simulink model "Simplified_TriPed"  (R2020a)
settings: Solver=VariableStepAuto  StartTime=0.0  StopTime=inf  RelTol=1e-3  EnableMultiTasking=on
values from neighbouring files (symbols this model uses):
  s = 1/(2*r)    [Weg0.m]
undefined symbols (not defined in the file or in its folder): sigbuilder_block, X, Y, Z
libraries: sm_lib x13, nesl_utility x4, ros2lib x3, powerlib_meascontrol x3, simulink x2, vrlib x1
(part 1 of 2)
settings Model: PacingRate=0.100000  OrderedModelArguments=off  Creator=maxde  LastModifiedBy=jan-b
settings DataIOCC: LimitDataPoints=on  MaxDataPoints=10000
settings OptimizationCC: LifeSpan=inf
settings DebuggingCC: AllowSymbolicDim=off  SFUnexpectedBacktrackingDiag=warning  SFNoUnconditionalDefaultTransitionDiag=warning  SFExecutionAtInitializationDiag=none  ArithmeticOperatorsInVariantConditions=warning
settings SFSimCC: SimUseLocalCustomCode=off  CustomCodeUndefinedFunction=UseInterfaceOnly
settings RTWCC: RTWUseLocalCustomCode=off
settings CodeAppCC: StateflowObjectComments=on
settings GRTTargetCC: TargetLangStandard=C89/C90 (ANSI)
settings ConfigComp: CovMetricSettings=dw  CovHtmlReporting=on  CovSaveCumulativeToWorkspaceVar=on  CovSaveSingleToWorkspaceVar=on  CovExternalEMLEnable=off  CovSFcnEnable=off
settings SimscapeCC: SimscapeLogType=all  SimscapeLogSimulationStatistics=on  SimscapeLogDataHistory=10000

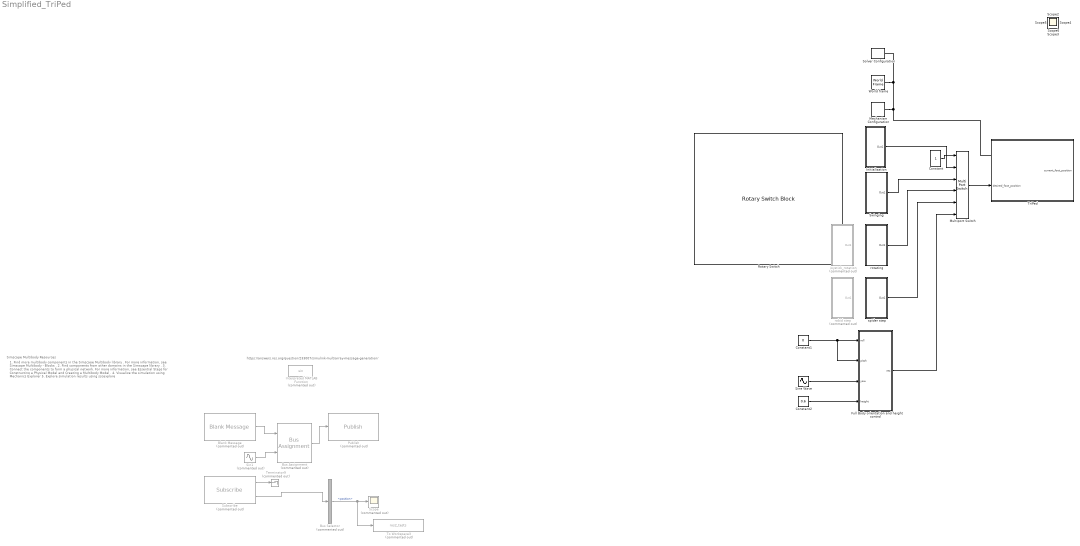
== system Simplified_TriPed ==
  note: https://answers.ros.org/question/233007/simulink-multiarray-message-generation/
  note: 1. Find more multibody components in the Simscape Multibody library .
      | For more information, see Simscape Multibody - Blocks .
      | 2. Find components from other domains in the Simscape library .
      | 3. Connect the components to form a physical network.
      | For more information, see Essential Steps for Constructing a Physical Model and Creating a Multibody Model .
      | 4. Visualize the simulation using Mechanics Explorer
      | 5. Explore simulation results using sscexplore
  note: Simscape Multibody Resources
  Blank Message : ros2lib/Blank Message  Commented=on  messageType=pendulum_msgs/JointState  SampleTime=inf
      settings: SourceProductBaseCode=RR
  Bus Assignment : BusAssignment  Commented=on  AssignedSignals=position
  Bus Selector : BusSelector  Commented=on  OutputSignals=position
  Constant : Constant
  Constant1 : Constant  Value=0
  Constant2 : Constant  Value=0.6
  Full Body orientation and height control : Subsystem
  Initialisation : Subsystem
  Interpreted MATLAB Function : MATLABFcn  Commented=on
  Mechanism Configuration : sm_lib/Utilities/Mechanism Configuration  UniformGravity=Constant  GravityVector=[0 0 -9.80665]  GravityUnits=m/s^2  LinearizationDelta=0.001
  Multiport Switch : MultiPortSwitch  Inputs=5
  Publish : ros2lib/Publish  Commented=on  topicSource=Specify your own  topic=/test_geometry  messageType=pendulum_msgs/JointState  QOSHistory=Keep last  QOSDepth=1  QOSReliability=Reliable  QOSDurability=Volatile
      settings: SourceProductBaseCode=RR
  Rotary Switch : RotarySwitchBlock
      settings: Values={{'Initialisation', 'Swinging', 'Rotating', 'Stepping', 'Full Body Kinematics'}, [1 2 3 4 5]}
  Scope : Scope  Commented=on
  Sin1 : Sin  Commented=on  Amplitude=pi/4  Frequency=2*pi/1  SampleTime=0.02
  Sine Wave : Sin  SampleTime=0
  Solver Configuration : nesl_utility/Solver Configuration  PhysicalDomain=network_engine_domain  SubClassName=solver  LeftPortType=input  RightPortType=generic  Tones=[]  Harmonics=[]  SimulateNoise=off  Profile=off  UseLocalSampling=off  EnableSwitchedLinearOptims=on  FrequencyDomain=off  UseCCode=off  RelTol=0.001  AbsTol=1e-06  MinStep=1e-09  ToWorkspace=off  RevertToSquareIcSolve=off  NumHomotopyIterations=100  PhasorMode=off  PhasorModeNumHarmonics=1  DoDC=off  ResidualTolerance=1e-09  UseLocalSolver=off  LocalSolverChoice=NE_BACKWARD_EULER_ADVANCER  LocalSolverSampleTime=0.001  DoFixedCost=off  MaxNonlinIter=3  MaxModeIter=2  LinearAlgebra=Sparse  EquationFormulation=NE_TIME_EF  DelaysMemoryBudget=1024  AutomaticFiltering=on  FilteringTimeConstant=0.001  PartitionStorageMethod=AS_NEEDED  PartitionMemoryBudget=1024  PartitionMethod=FAST
      settings: SourceProductBaseCode=MT,SS
  Subscribe : ros2lib/Subscribe  Commented=on  topicSource=Specify your own  topic=/test_geometry  messageType=pendulum_msgs/JointState  sampleTime=-1  QOSHistory=Keep last  QOSDepth=1  QOSReliability=Reliable  QOSDurability=Volatile
      settings: SourceProductBaseCode=RR
  Swinging : Subsystem
  Terminator9 : Terminator  Commented=on
  To Workspace3 : ToWorkspace  Commented=on  VariableName=ros2_tests  SaveFormat=Timeseries  SampleTime=-1
  TriPed : Subsystem
      settings: PortSchema="{\"entries\":[{\"content\":{\"sides\":[{\"content\":{\"connectorIds\":[\"LConn1\",\"In1\"]},\"type\":\"ConnectorPlacement.EquallySpacedRectSide\",\"uuid\":\"cf937cc4-9946-458f-a00c-c6b64d50e5dd\"},{\"content\":{\"connectorIds\":[\"Out1\"],\"side\":\"RIGHT\"},\"type\":\"ConnectorPlacement.EquallySpacedRectSide\",\"uuid\":\"24e17f8e-a145-44bf-b20e-4a80bbb5751f\"},{\"content\":{\"connectorIds\":[],\"side\":\"TOP\"},\"type\":\"ConnectorPlacement.EquallySpacedRectSide\",\"uuid\":\"6e43fe6c-017a-4e02-a518-41141b50f8f7\"}]},\"type\":\"ConnectorPlacement.EquallySpacedConnector\",\"uuid\":\"8dc904d1-a5ef-4597-b7a1-5eba3e01f89e\"}],\"packageUris\":[\"http://schema.mathworks.com/mf0/Connector/19700101\"],\"version\":\"1.0\"}"
      mask Display: image('./icons/triped_complete_view.png')
  World frame : sm_lib/Frames and Transforms/World Frame
  joystick_rotation : Subsystem  Commented=on
  rabid step : Subsystem  Commented=on
  rotating : Subsystem
  spider step : Subsystem
  Scope{1..6} (6 alike) : Scope
  wires:
  Blank Message/1 -> Bus Assignment/1
  Bus Assignment/1 -> Publish/1
  Sin1/1 -> Bus Assignment/2
  Subscribe/1 -> Terminator9/1
  Subscribe/2 -> Bus Selector/1
  Bus Selector/1 -> Scope/1, To Workspace3/1  "<position>"
  Sine Wave/1 -> Full Body orientation and height control/3(yaw)
  rotating/1(Out1) -> Multiport Switch/4
  Full Body orientation and height control/1(res) -> Multiport Switch/6
  Constant/1 -> Multiport Switch/1
  Swinging/1(Out1) -> Multiport Switch/3
  Initialisation/1(Out1) -> Multiport Switch/2
  spider step/1(Out1) -> Multiport Switch/5
  Constant1/1 -> Full Body orientation and height control/2(pitch), Full Body orientation and height control/1(roll)
  Constant2/1 -> Full Body orientation and height control/4(height)
  Multiport Switch/1 -> TriPed/1(desired_foot_position)
  connections:
  Mechanism Configuration/RConn1 -- Solver Configuration/RConn1 -- World frame/RConn1 -- TriPed/LConn1

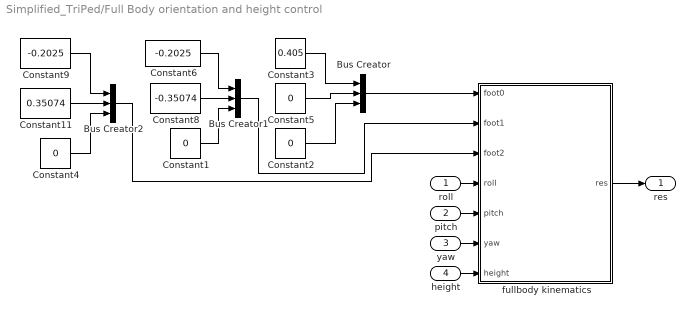
== system Simplified_TriPed/Full Body orientation and height control ==
  roll : Inport
  pitch : Inport  Port=2
  yaw : Inport  Port=3
  height : Inport  Port=4
  Bus Creator : BusCreator  Inputs=3
  Bus Creator1 : BusCreator  Inputs=3
  Bus Creator2 : BusCreator  Inputs=3
  Constant{1..2,4..5} (4 alike) : Constant  Value=0
  Constant11 : Constant  Value=0.35074
  Constant3 : Constant  Value=0.405
  Constant6 : Constant  Value=-0.2025
  Constant8 : Constant  Value=-0.35074
  Constant9 : Constant  Value=-0.2025
  fullbody kinematics : MATLAB Function  TreatAsAtomicUnit=on
  res : Outport
  wires:
  Bus Creator2/1 -> fullbody kinematics/3(foot2)
  pitch/1 -> fullbody kinematics/5(pitch)
  roll/1 -> fullbody kinematics/4(roll)
  height/1 -> fullbody kinematics/7(height)
  fullbody kinematics/1(res) -> res/1
  Bus Creator/1 -> fullbody kinematics/1(foot0)
  Bus Creator1/1 -> fullbody kinematics/2(foot1)
  yaw/1 -> fullbody kinematics/6(yaw)
  Constant5/1 -> Bus Creator/2
  Constant3/1 -> Bus Creator/1
  Constant2/1 -> Bus Creator/3
  Constant8/1 -> Bus Creator1/2
  Constant6/1 -> Bus Creator1/1
  Constant1/1 -> Bus Creator1/3
  Constant11/1 -> Bus Creator2/2
  Constant9/1 -> Bus Creator2/1
  Constant4/1 -> Bus Creator2/3

== system Simplified_TriPed/Initialisation ==
  note: Initialisation
  note: Initialiszes the system to a height of 60 cm above ground
  Bus Creator1 : BusCreator  Inputs=9
  Constant11 : Constant  Value=0.35074
  Constant3 : Constant  Value=0.405
  Constant5 : Constant  Value=0
  Constant6 : Constant  Value=-0.2025
  Constant8 : Constant  Value=-0.35074
  Constant9 : Constant  Value=-0.2025
  Ramp : simulink/Sources/Ramp  slope=-0.3  start=0  InitialOutput=-0.023  VectorParams1D=off
  Saturation : Saturate  LowerLimit=-0.6
  Out1 : Outport
  wires:
  Constant9/1 -> Bus Creator1/7
  Constant5/1 -> Bus Creator1/2
  Constant6/1 -> Bus Creator1/4
  Constant3/1 -> Bus Creator1/1
  Saturation/1 -> Bus Creator1/3, Bus Creator1/6, Bus Creator1/9
  Constant8/1 -> Bus Creator1/5
  Constant11/1 -> Bus Creator1/8
  Bus Creator1/1 -> Out1/1
  Ramp/1 -> Saturation/1

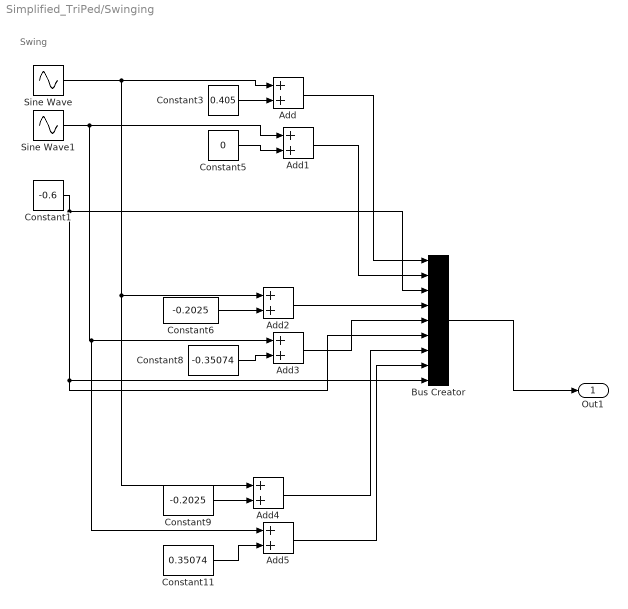
== system Simplified_TriPed/Swinging ==
  note: Swing
  Add{,1..5} (6 alike) : Sum
  Bus Creator : BusCreator  Inputs=9
  Constant1 : Constant  Value=-0.6
  Constant11 : Constant  Value=0.35074
  Constant3 : Constant  Value=0.405
  Constant5 : Constant  Value=0
  Constant6 : Constant  Value=-0.2025
  Constant8 : Constant  Value=-0.35074
  Constant9 : Constant  Value=-0.2025
  Sine Wave : Sin  Amplitude=0.1  Frequency=pi  SampleTime=0
  Sine Wave1 : Sin  Amplitude=0.1  Frequency=pi  Phase=pi/2  SampleTime=0
  Out1 : Outport
  wires:
  Add1/1 -> Bus Creator/2
  Add4/1 -> Bus Creator/7
  Add3/1 -> Bus Creator/5
  Constant1/1 -> Bus Creator/3, Bus Creator/6, Bus Creator/9
  Add/1 -> Bus Creator/1
  Add5/1 -> Bus Creator/8
  Add2/1 -> Bus Creator/4
  Bus Creator/1 -> Out1/1
  Constant6/1 -> Add2/2
  Constant8/1 -> Add3/2
  Constant9/1 -> Add4/2
  Constant5/1 -> Add1/2
  Sine Wave/1 -> Add4/1, Add2/1, Add/1
  Constant11/1 -> Add5/2
  Constant3/1 -> Add/2
  Sine Wave1/1 -> Add5/1, Add3/1, Add1/1

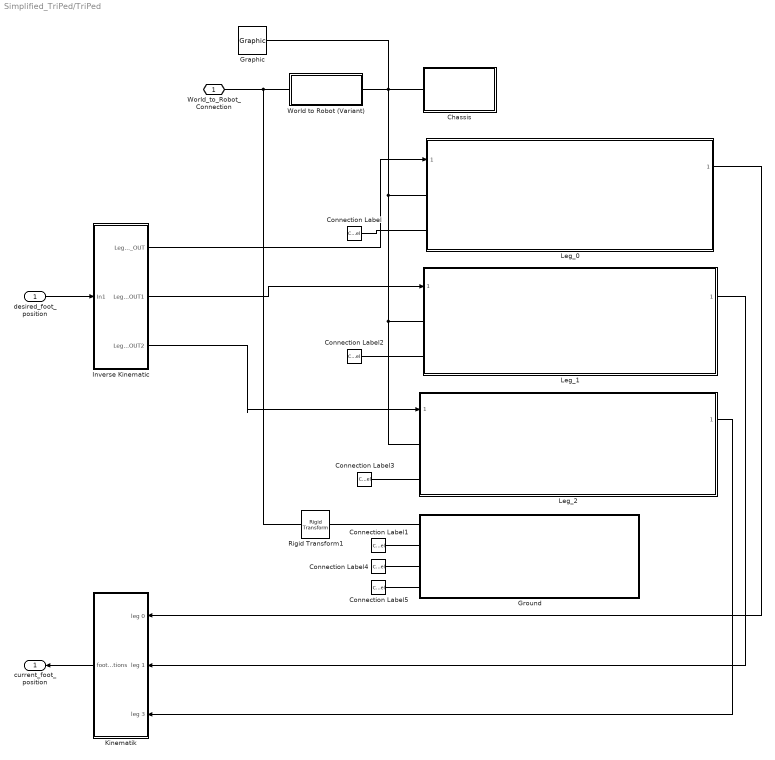
== system Simplified_TriPed/TriPed ==
  desired_foot_position : Inport
  Chassis : Subsystem
  Connection Label : ConnectionLabel  Label=leg0_GroundForce_Connection
  Connection Label1 : ConnectionLabel  Label=leg0_GroundForce_Connection
  Connection Label2 : ConnectionLabel  Label=leg1_GroundForce_Connection
  Connection Label3 : ConnectionLabel  Label=leg2_GroundForce_Connection
  Connection Label4 : ConnectionLabel  Label=leg1_GroundForce_Connection
  Connection Label5 : ConnectionLabel  Label=leg2_GroundForce_Connection
  Graphic : sm_lib/Body Elements/Graphic  GraphicType=Marker  MarkerShape=Frame  MarkerSize=40  GraphicVisPropType=SimpleVisualProperties  GraphicDiffuseColor=[0.0 1.0 0.0]  GraphicSpecularColor=[0.5 0.5 0.5 1.0]  GraphicAmbientColor=[0.15 0.15 0.15 1.0]  GraphicEmissiveColor=[0.0 0.0 0.0 1.0]  GraphicShininess=75  GraphicOpacity=1.0
  Ground : Subsystem
  Inverse Kinematic : Subsystem
  Kinematik : Subsystem
      settings: PortSchema="{\"entries\":[{\"content\":{\"sides\":[{\"content\":{\"connectorIds\":[\"Out1\"]},\"type\":\"ConnectorPlacement.EquallySpacedRectSide\",\"uuid\":\"723aa903-851a-4664-882b-cb687275721b\"},{\"content\":{\"connectorIds\":[\"In1\",\"In2\",\"In3\"],\"side\":\"RIGHT\"},\"type\":\"ConnectorPlacement.EquallySpacedRectSide\",\"uuid\":\"f9e95ccf-8a42-4456-81db-8f425e241ec1\"},{\"content\":{\"connectorIds\":[],\"side\":\"TOP\"},\"type\":\"ConnectorPlacement.EquallySpacedRectSide\",\"uuid\":\"175b5798-3047-4472-9bca-bb6c2911fede\"}]},\"type\":\"ConnectorPlacement.EquallySpacedConnector\",\"uuid\":\"62df2873-5e03-4e99-98e6-e4829089aed6\"}],\"packageUris\":[\"http://schema.mathworks.com/mf0/Connector/19700101\"],\"version\":\"1.0\"}"
  Leg_0 : Subsystem  ReferencedSubsystem=Simplified_Leg_Assembly  LegNumber=0
  Leg_1 : Subsystem  ReferencedSubsystem=Simplified_Leg_Assembly  LegNumber=1
  Leg_2 : Subsystem  ReferencedSubsystem=Simplified_Leg_Assembly  LegNumber=2
  Rigid Transform1 : sm_lib/Frames and Transforms/Rigid Transform  TranslationMethod=StandardAxis  TranslationStandardOffset=-0.3  TranslationLengthUnit=m  TranslationStandardAxis=+Z  TranslationCartesianOffset=[0 0 0]  TranslationROffset=0  TranslationROffsetUnits=m  TranslationZOffset=0  TranslationZOffsetUnits=m  TranslationThetaOffset=0  TranslationThetaOffsetUnits=deg  RotationMethod=None  RotationAngleUnits=deg  RotationStandardAxis=+Z  RotationAngle=0.0  RotationArbitraryAxis=[0 0 1]  FollAlignAxisA=+X  BaseAlignAxisA=+Y  FollAlignAxisB=+Y  BaseAlignAxisB=+Z  RotationSequenceAxes=FollowerAxes  RotationSequence=XYX  RotationSequenceAngles=[0 0 0]  RotationSequenceAnglesUnits=deg  RotationMatrix=[1 0 0; 0 1 0; 0 0 1]
  World to Robot (Variant) : Subsystem  Variant=on  VariantControlMode=Label  LabelModeActiveChoice=Choice_2
  World_to_Robot_Connection : PMIOPort  Side=Left
  current_foot_position : Outport
  wires:
  Inverse Kinematic/1(Leg0Bus_OUT) -> Leg_0/1
  Inverse Kinematic/2(Leg0Bus_OUT1) -> Leg_1/1
  Inverse Kinematic/3(Leg0Bus_OUT2) -> Leg_2/1
  desired_foot_position/1 -> Inverse Kinematic/1(In1)
  Leg_0/1 -> Kinematik/1(leg 0)
  Leg_1/1 -> Kinematik/2(leg 1)
  Leg_2/1 -> Kinematik/3(leg 3)
  Kinematik/1(foot positions) -> current_foot_position/1
  connections:
  Connection Label4/LConn1 -- Ground/LConn3
  Ground/LConn4 -- Connection Label5/LConn1
  Connection Label1/LConn1 -- Ground/LConn2
  World to Robot (Variant)/LConn1 -- Rigid Transform1/LConn1 -- World_to_Robot_Connection/RConn1
  Leg_2/LConn1 -- World to Robot (Variant)/RConn1 -- Graphic/RConn1 -- Chassis/LConn1 -- Leg_0/LConn1 -- Leg_1/LConn1
  Connection Label/LConn1 -- Leg_0/LConn2
  Connection Label2/LConn1 -- Leg_1/LConn2
  Connection Label3/LConn1 -- Leg_2/LConn2
  Ground/LConn1 -- Rigid Transform1/RConn1

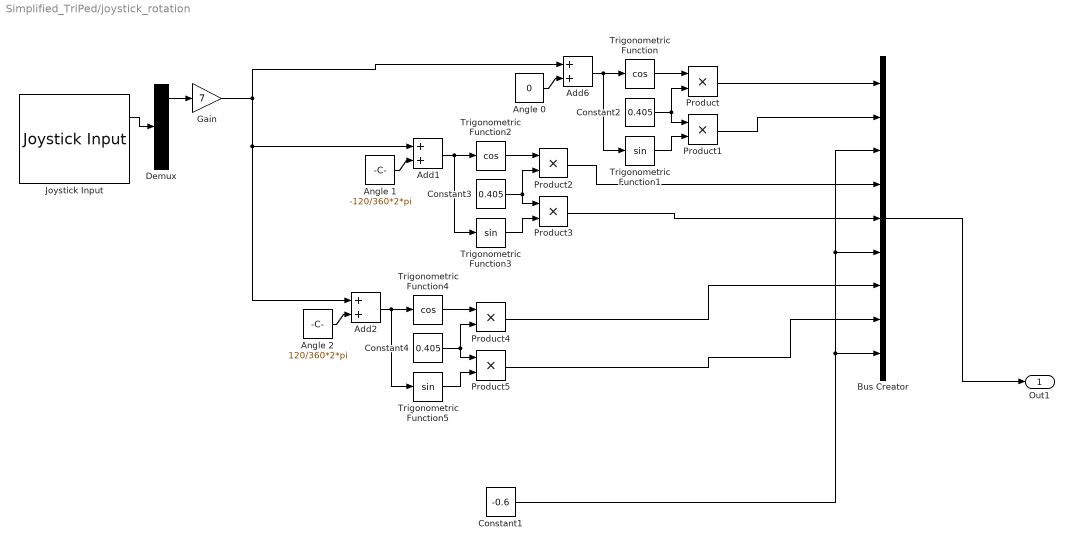
== system Simplified_TriPed/joystick_rotation ==
  Add1 : Sum
  Add2 : Sum
  Add6 : Sum
  Angle 0 : Constant  Value=0
  Angle 1 : Constant  Value=-120/360*2*pi
  Angle 2 : Constant  Value=120/360*2*pi
  Bus Creator : BusCreator  Inputs=9
  Constant1 : Constant  Value=-0.6
  Constant2 : Constant  Value=0.405
  Constant3 : Constant  Value=0.405
  Constant4 : Constant  Value=0.405
  Demux : Demux  Outputs=5
  Gain : Gain  Gain=7
  Joystick Input : vrlib/Joystick Input  joyid=1  adjustports=on  forcefeed=off
  Product{,1..5} (6 alike) : Product
  Trigonometric Function : Trigonometry  Operator=cos
  Trigonometric Function1 : Trigonometry
  Trigonometric Function2 : Trigonometry  Operator=cos
  Trigonometric Function3 : Trigonometry
  Trigonometric Function4 : Trigonometry  Operator=cos
  Trigonometric Function5 : Trigonometry
  Out1 : Outport
  wires:
  Constant1/1 -> Bus Creator/3, Bus Creator/6, Bus Creator/9
  Bus Creator/1 -> Out1/1
  Angle 0/1 -> Add6/2
  Add6/1 -> Trigonometric Function1/1, Trigonometric Function/1
  Trigonometric Function/1 -> Product/1
  Constant2/1 -> Product/2, Product1/1
  Trigonometric Function1/1 -> Product1/2
  Product/1 -> Bus Creator/1
  Product1/1 -> Bus Creator/2
  Constant3/1 -> Product2/2, Product3/1
  Trigonometric Function3/1 -> Product3/2
  Trigonometric Function2/1 -> Product2/1
  Angle 1/1 -> Add1/2
  Add1/1 -> Trigonometric Function3/1, Trigonometric Function2/1
  Product2/1 -> Bus Creator/4
  Product3/1 -> Bus Creator/5
  Add2/1 -> Trigonometric Function5/1, Trigonometric Function4/1
  Angle 2/1 -> Add2/2
  Demux/1 -> Gain/1
  Trigonometric Function5/1 -> Product5/2
  Trigonometric Function4/1 -> Product4/1
  Constant4/1 -> Product4/2, Product5/1
  Product4/1 -> Bus Creator/7
  Product5/1 -> Bus Creator/8
  Joystick Input/1 -> Demux/1
  Gain/1 -> Add2/1, Add1/1, Add6/1

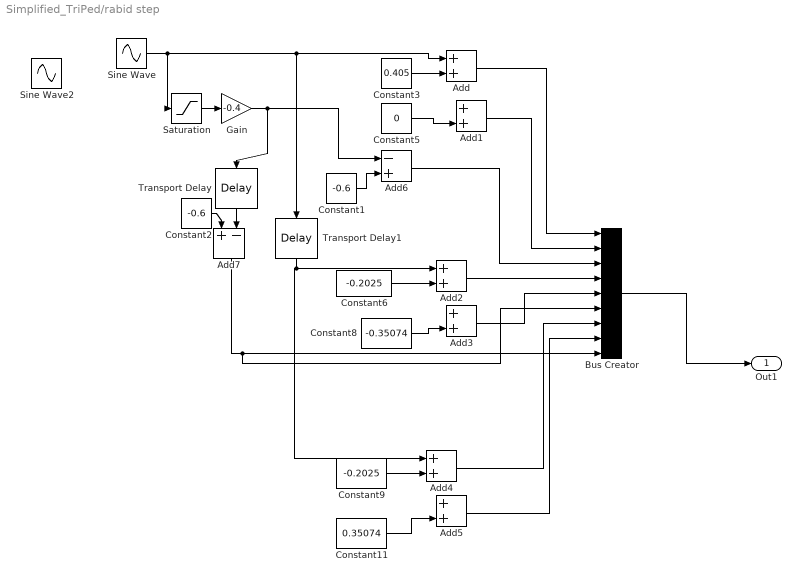
== system Simplified_TriPed/rabid step ==
  Add{,1..5} (6 alike) : Sum
  Add6 : Sum  Inputs=-+
  Add7 : Sum  Inputs=+-
  Bus Creator : BusCreator  Inputs=9
  Constant1 : Constant  Value=-0.6
  Constant11 : Constant  Value=0.35074
  Constant2 : Constant  Value=-0.6
  Constant3 : Constant  Value=0.405
  Constant5 : Constant  Value=0
  Constant6 : Constant  Value=-0.2025
  Constant8 : Constant  Value=-0.35074
  Constant9 : Constant  Value=-0.2025
  Gain : Gain  Gain=-0.4
  Saturation : Saturate  UpperLimit=10  LowerLimit=0
  Sine Wave : Sin  Amplitude=0.2  Frequency=pi  SampleTime=0
  Sine Wave2 : Sin  Amplitude=0.2  Frequency=pi  SampleTime=0
  Transport Delay : TransportDelay  DelayTime=0.25
  Transport Delay1 : TransportDelay  DelayTime=0.25
  Out1 : Outport
  wires:
  Add1/1 -> Bus Creator/2
  Add4/1 -> Bus Creator/7
  Add3/1 -> Bus Creator/5
  Add/1 -> Bus Creator/1
  Add5/1 -> Bus Creator/8
  Add2/1 -> Bus Creator/4
  Bus Creator/1 -> Out1/1
  Constant6/1 -> Add2/2
  Constant8/1 -> Add3/2
  Constant9/1 -> Add4/2
  Constant5/1 -> Add1/2
  Sine Wave/1 -> Saturation/1, Transport Delay1/1, Add/1
  Constant11/1 -> Add5/2
  Constant3/1 -> Add/2
  Saturation/1 -> Gain/1
  Constant1/1 -> Add6/2
  Add7/1 -> Bus Creator/6, Bus Creator/9
  Transport Delay1/1 -> Add4/1, Add2/1
  Add6/1 -> Bus Creator/3
  Transport Delay/1 -> Add7/2
  Constant2/1 -> Add7/1
  Gain/1 -> Add6/1, Transport Delay/1

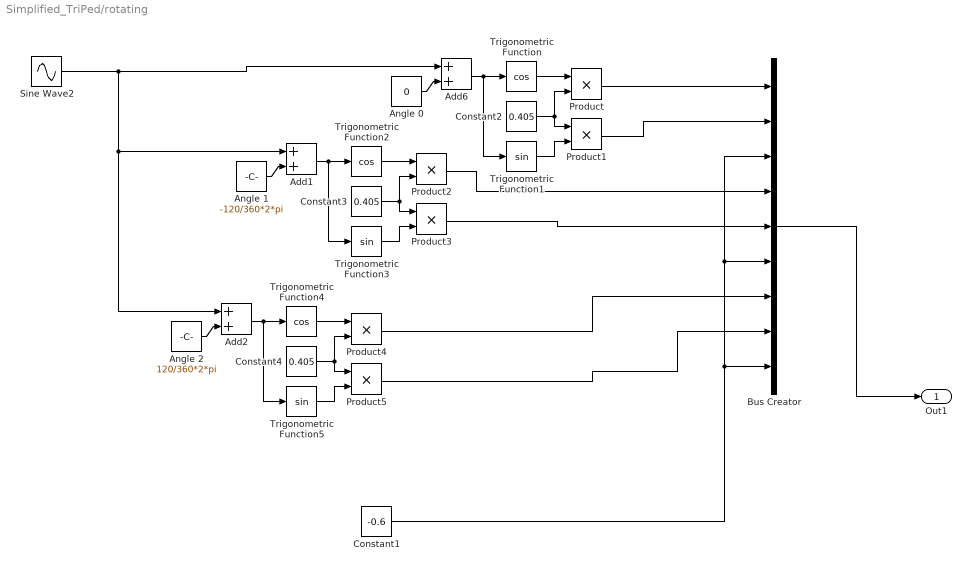
== system Simplified_TriPed/rotating ==
  Add1 : Sum
  Add2 : Sum
  Add6 : Sum
  Angle 0 : Constant  Value=0
  Angle 1 : Constant  Value=-120/360*2*pi
  Angle 2 : Constant  Value=120/360*2*pi
  Bus Creator : BusCreator  Inputs=9
  Constant1 : Constant  Value=-0.6
  Constant2 : Constant  Value=0.405
  Constant3 : Constant  Value=0.405
  Constant4 : Constant  Value=0.405
  Product{,1..5} (6 alike) : Product
  Sine Wave2 : Sin  Frequency=pi  SampleTime=0
  Trigonometric Function : Trigonometry  Operator=cos
  Trigonometric Function1 : Trigonometry
  Trigonometric Function2 : Trigonometry  Operator=cos
  Trigonometric Function3 : Trigonometry
  Trigonometric Function4 : Trigonometry  Operator=cos
  Trigonometric Function5 : Trigonometry
  Out1 : Outport
  wires:
  Constant1/1 -> Bus Creator/3, Bus Creator/6, Bus Creator/9
  Bus Creator/1 -> Out1/1
  Angle 0/1 -> Add6/2
  Add6/1 -> Trigonometric Function1/1, Trigonometric Function/1
  Trigonometric Function/1 -> Product/1
  Constant2/1 -> Product/2, Product1/1
  Trigonometric Function1/1 -> Product1/2
  Product/1 -> Bus Creator/1
  Product1/1 -> Bus Creator/2
  Constant3/1 -> Product2/2, Product3/1
  Trigonometric Function3/1 -> Product3/2
  Trigonometric Function2/1 -> Product2/1
  Angle 1/1 -> Add1/2
  Add1/1 -> Trigonometric Function3/1, Trigonometric Function2/1
  Product2/1 -> Bus Creator/4
  Product3/1 -> Bus Creator/5
  Add2/1 -> Trigonometric Function5/1, Trigonometric Function4/1
  Angle 2/1 -> Add2/2
  Sine Wave2/1 -> Add2/1, Add1/1, Add6/1
  Trigonometric Function5/1 -> Product5/2
  Trigonometric Function4/1 -> Product4/1
  Constant4/1 -> Product4/2, Product5/1
  Product4/1 -> Bus Creator/7
  Product5/1 -> Bus Creator/8

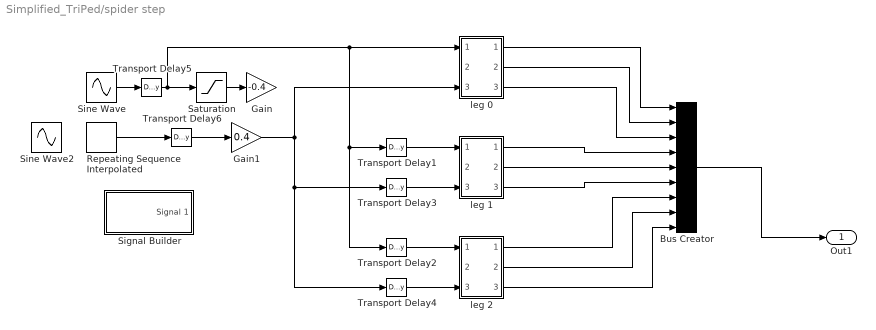
== system Simplified_TriPed/spider step ==
  Bus Creator : BusCreator  Inputs=9
  Gain : Gain  Gain=-0.4
  Gain1 : Gain  Gain=0.4
  Repeating Sequence Interpolated : simulink/Sources/Repeating Sequence Interpolated  OutValues=[0 0.3 0.3 0.1 0.03 0.005 0.001 0].'  TimeValues="[0 0.2 0.5 0.6 0.8 0.9  0.95 1].'"  LookUpMeth=Interpolation-Use End Values  tsamp=0.01  OutMin=[]  OutMax=[]  OutDataTypeStr=double  OutputDataTypeScalingMode=double  OutDataType=fixdt(0,8)  OutScaling=2^-10
  Saturation : Saturate  UpperLimit=10  LowerLimit=0
  Signal Builder : Subsystem  Tag=STV Subsys  LoadFcn=sigbuilder_block('load');  StartFcn=sigbuilder_block('start');  StopFcn=sigbuilder_block('stop');  ClipboardFcn=sigbuilder_block('clipboard');  mask(Sigbuilder block){tuvar=[0:10]}
      mask help: Simulink:masks:SigbuilderBlock_MD
      mask init:
      | if ~strcmp(get_param(bdroot(gcbh),'SimulationStatus'),'stopped') tuvar = sigbuilder_block('maskInit'); end
      settings: CopyFcn=sigbuilder_block('copy');  DeleteFcn=sigbuilder_block('delete');  ModelCloseFcn=sigbuilder_block('modelClose');  PreSaveFcn=sigbuilder_block('preSave');  PauseFcn=sigbuilder_block('pause');  ContinueFcn=sigbuilder_block('continue');  NameChangeFcn=sigbuilder_block('namechange');  OpenFcn=sigbuilder_block('open',[437.6 199.2 550.4 400 ]);  CloseFcn=sigbuilder_block('close');
      mask Display: plot(0, 0, 100, 100,[2, 2, 32, 32, 2], [68, 8, 8, 68, 68],[32, 2], [38, 38], [32, 19, 2],[53, 60, 44], [32, 17, 17, 2],[16, 16, 31, 31]);txt = getActiveGroup(gcbh);text(2, 100, txt,'verticalAlignment', 'top');
  Sine Wave : Sin  Amplitude=0.2  Frequency=pi  SampleTime=0
  Sine Wave2 : Sin  Amplitude=0.2  Frequency=pi  SampleTime=0
  Transport Delay1 : TransportDelay  DelayTime=0.33
  Transport Delay2 : TransportDelay  DelayTime=0.66
  Transport Delay3 : TransportDelay  DelayTime=0.33
  Transport Delay4 : TransportDelay  DelayTime=0.66
  Transport Delay5 : TransportDelay  DelayTime=0.3
  Transport Delay6 : TransportDelay  DelayTime=0.3
  leg 0 : Subsystem
  leg 1 : Subsystem
  leg 2 : Subsystem
  Out1 : Outport
  wires:
  Bus Creator/1 -> Out1/1
  Sine Wave/1 -> Transport Delay5/1
  Saturation/1 -> Gain/1
  Repeating Sequence Interpolated/1 -> Transport Delay6/1
  leg 0/1(Out1) -> Bus Creator/1
  leg 0/2(Out2) -> Bus Creator/2
  leg 0/3(Out3) -> Bus Creator/3
  leg 1/1(Out1) -> Bus Creator/4
  leg 1/2(Out2) -> Bus Creator/5
  leg 1/3(Out3) -> Bus Creator/6
  leg 2/1(Out1) -> Bus Creator/7
  leg 2/2(Out2) -> Bus Creator/8
  leg 2/3(Out3) -> Bus Creator/9
  Transport Delay1/1 -> leg 1/1(In1)
  Transport Delay3/1 -> leg 1/3(In3)
  Transport Delay4/1 -> leg 2/3(In3)
  Transport Delay2/1 -> leg 2/1(In1)
  Transport Delay5/1 -> Transport Delay2/1, Transport Delay1/1, leg 0/1(In1), Saturation/1
  Transport Delay6/1 -> Gain1/1
  Gain1/1 -> Transport Delay4/1, Transport Delay3/1, leg 0/3(In3)

== system Simplified_TriPed/TriPed/Chassis ==
  Chassis : sm_lib/Body Elements/File Solid  ExtGeomFileName=./triped-files/TriPed_Chassis_überarbeitet.stl  UnitType=Custom  ExtGeomFileUnits=mm  StepReaderType=HEX  ExportConvexHullGeometry=off  InertiaType=Custom  Mass=9.273  MassUnits=kg  CenterOfMass=[0 0 10.44]  CenterOfMassUnits=mm  MomentsOfInertia=[0.121 0.121 0.199]  MomentsOfInertiaUnits=kg*m^2  ProductsOfInertia=[0 0 0]  ProductsOfInertiaUnits=kg*m^2  BasedOnType=DensityFromFile  Density=1000  DensityUnits=kg/m^3  DoExposeReferenceFrame=on  SerializedFrames=<Frames/>  GraphicType=FromGeometry  MarkerShape=Sphere  MarkerSize=10  GraphicVisPropType=SimpleVisualProperties  GraphicDiffuseColor=[0.5 0.5 0.5]  GraphicSpecularColor=[0.5 0.5 0.5 1.0]  GraphicAmbientColor=[0.15 0.15 0.15 1.0]  GraphicEmissiveColor=[0.0 0.0 0.0 1.0]  GraphicShininess=75  GraphicOpacity=1
  " Chassis_connection" : PMIOPort  Side=Left
  connections:
  Chassis/RConn1 -- " Chassis_connection"/RConn1

== system Simplified_TriPed/TriPed/Ground ==
  Goto : Goto  Commented=on  GotoTag=leg0_groundForce  TagVisibility=global
  Goto1 : Goto  Commented=on  GotoTag=leg1_groundForce  TagVisibility=global
  Goto2 : Goto  Commented=on  GotoTag=leg2_groundForce  TagVisibility=global
  Ground : sm_lib/Body Elements/Brick Solid  GraphicAmbientColor=[0.15 0.15 0.15 1.0]  BasedOnType=Density  BrickDimensions=[4 4 0.1]  BrickDimensionUnits=m  CenterOfMass=[0 0 0]  CenterOfMassUnits=m  GraphicDiffuseColor=[0.4 0.2 0.0]  Density=1000  DensityUnits=kg/m^3  DoExposeReferenceFrame=on  GraphicEmissiveColor=[0.0 0.0 0.0 1.0]  ExportEntireGeometry=on  SerializedFrames=<Frames/>  MarkerShape=Sphere  MarkerSize=10  GraphicType=FromGeometry  InertiaType=CalculateFromGeometry  Mass=1  MassUnits=kg  MomentsOfInertia=[1 1 1]  MomentsOfInertiaUnits=kg*m^2  GraphicOpacity=0.8  ProductsOfInertia=[0 0 0]  ProductsOfInertiaUnits=kg*m^2  GraphicShininess=75  GraphicSpecularColor=[0.5 0.5 0.5 1.0]  GraphicVisPropType=SimpleVisualProperties
  Quantise_Leg_Forces : Subsystem
  SpatialContactForce-Leg0 : sm_lib/Forces and Torques/Spatial Contact Force  CoefficientOfDynamicFriction=0.3  CoefficientOfStaticFriction=0.5  NormalDamping=1e4  NormalDampingUnits=N/(m/s)  NormalStiffness=1e6  NormalStiffnessUnits=N/m  FrictionalCriticalVelocity=1e-3  FrictionalCriticalVelocityUnits=m/s  ZeroCrossDetectContactStartAndEnd=on  SenseFrictionalForceMagnitude=off  SenseNormalForceMagnitude=on  SenseSeparationDistance=off  NormalTransitionRegionWidth=1e-4  NormalTransitionRegionWidthUnits=m  FrictionType=SmoothStickSlip
  SpatialContactForce-Leg1 : sm_lib/Forces and Torques/Spatial Contact Force  CoefficientOfDynamicFriction=0.3  CoefficientOfStaticFriction=0.5  NormalDamping=1e4  NormalDampingUnits=N/(m/s)  NormalStiffness=1e6  NormalStiffnessUnits=N/m  FrictionalCriticalVelocity=1e-3  FrictionalCriticalVelocityUnits=m/s  ZeroCrossDetectContactStartAndEnd=on  SenseFrictionalForceMagnitude=off  SenseNormalForceMagnitude=on  SenseSeparationDistance=off  NormalTransitionRegionWidth=1e-4  NormalTransitionRegionWidthUnits=m  FrictionType=SmoothStickSlip
  SpatialContactForce-Leg2 : sm_lib/Forces and Torques/Spatial Contact Force  CoefficientOfDynamicFriction=0.3  CoefficientOfStaticFriction=0.5  NormalDamping=1e4  NormalDampingUnits=N/(m/s)  NormalStiffness=1e6  NormalStiffnessUnits=N/m  FrictionalCriticalVelocity=1e-3  FrictionalCriticalVelocityUnits=m/s  ZeroCrossDetectContactStartAndEnd=on  SenseFrictionalForceMagnitude=off  SenseNormalForceMagnitude=on  SenseSeparationDistance=off  NormalTransitionRegionWidth=1e-4  NormalTransitionRegionWidthUnits=m  FrictionType=SmoothStickSlip
  World_to_Ground : sm_lib/Frames and Transforms/Rigid Transform  TranslationMethod=Cartesian  TranslationStandardOffset=0  TranslationLengthUnit=m  TranslationStandardAxis=+Z  TranslationCartesianOffset=[0 0 -0.5]  TranslationROffset=0  TranslationROffsetUnits=m  TranslationZOffset=0  TranslationZOffsetUnits=m  TranslationThetaOffset=0  TranslationThetaOffsetUnits=deg  RotationMethod=None  RotationAngleUnits=deg  RotationStandardAxis=+Z  RotationAngle=0.0  RotationArbitraryAxis=[0 0 1]  FollAlignAxisA=+X  BaseAlignAxisA=+Y  FollAlignAxisB=+Y  BaseAlignAxisB=+Z  RotationSequenceAxes=FollowerAxes  RotationSequence=XYX  RotationSequenceAngles=[0 0 0]  RotationSequenceAnglesUnits=deg  RotationMatrix=[1 0 0; 0 1 0; 0 0 1]
  World_to_Ground_2 : sm_lib/Joints/Weld Joint  JointMode=Normal  SenseConstraintForce=off  SenseConstraintForceX=off  SenseConstraintForceY=off  SenseConstraintForceZ=off  SenseConstraintTorque=off  SenseConstraintTorqueX=off  SenseConstraintTorqueY=off  SenseConstraintTorqueZ=off  SenseTotalForce=off  SenseTotalForceX=off  SenseTotalForceY=off  SenseTotalForceZ=off  SenseTotalTorque=off  SenseTotalTorqueX=off  SenseTotalTorqueY=off  SenseTotalTorqueZ=off  CompositeWrenchDir=FollowerOnBase  CompositeWrenchFrame=BaseFrame
  World_to_Ground1 : PMIOPort  Side=Left
  Force_GND_to_Leg_0 : PMIOPort  Port=2  Side=Left
  Force_GND_to_Leg_1 : PMIOPort  Port=3  Side=Left
  Force_GND_to_Leg_2 : PMIOPort  Port=4  Side=Left
  wires:
  Quantise_Leg_Forces/1(Out1) -> Goto/1
  Quantise_Leg_Forces/2(Out2) -> Goto1/1
  Quantise_Leg_Forces/3(Out3) -> Goto2/1
  connections:
  Ground/RConn1 -- World_to_Ground_2/RConn1
  Ground/LConn1 -- SpatialContactForce-Leg0/LConn1 -- SpatialContactForce-Leg1/LConn1 -- SpatialContactForce-Leg2/LConn1
  SpatialContactForce-Leg1/RConn1 -- Force_GND_to_Leg_1/RConn1
  World_to_Ground/LConn1 -- World_to_Ground1/RConn1
  SpatialContactForce-Leg2/RConn1 -- Force_GND_to_Leg_2/RConn1
  SpatialContactForce-Leg0/RConn1 -- Force_GND_to_Leg_0/RConn1
  World_to_Ground_2/LConn1 -- World_to_Ground/RConn1
  Quantise_Leg_Forces/LConn2 -- SpatialContactForce-Leg1/RConn2
  Quantise_Leg_Forces/LConn3 -- SpatialContactForce-Leg2/RConn2
  SpatialContactForce-Leg0/RConn2 -- Quantise_Leg_Forces/LConn1

== system Simplified_TriPed/TriPed/Inverse Kinematic ==
  In1 : Inport
  Constant : Constant  Value=0
  Constant1 : Constant
  Constant2 : Constant  Value=2
  Demux : Demux  Outputs=9
  Subsystem : Subsystem
  Subsystem1 : Subsystem
  Subsystem2 : Subsystem
  Leg0Bus_OUT : Outport
  Leg0Bus_OUT1 : Outport  Port=2
  Leg0Bus_OUT2 : Outport  Port=3
  wires:
  Demux/7 -> Subsystem2/1(x)
  Constant1/1 -> Subsystem1/4(LegNumber)
  Demux/9 -> Subsystem2/3(z)
  Constant/1 -> Subsystem/4(LegNumber)
  Constant2/1 -> Subsystem2/4(LegNumber)
  Demux/5 -> Subsystem1/2(y)
  Subsystem2/1(Leg0Bus_OUT) -> Leg0Bus_OUT2/1
  Demux/4 -> Subsystem1/1(x)
  Demux/1 -> Subsystem/1(x)
  Demux/6 -> Subsystem1/3(z)
  Demux/3 -> Subsystem/3(z)
  Demux/8 -> Subsystem2/2(y)
  Demux/2 -> Subsystem/2(y)
  Subsystem/1(Leg0Bus_OUT) -> Leg0Bus_OUT/1
  Subsystem1/1(Leg0Bus_OUT) -> Leg0Bus_OUT1/1
  In1/1 -> Demux/1

== system Simplified_TriPed/TriPed/Kinematik ==
  leg 0 : Inport
  leg 1 : Inport  Port=2
  leg 3 : Inport  Port=3
  MATLAB Function : MATLAB Function  TreatAsAtomicUnit=on
  foot positions : Outport
  wires:
  leg 0/1 -> MATLAB Function/1(leg_0)
  leg 1/1 -> MATLAB Function/2(leg_1)
  leg 3/1 -> MATLAB Function/3(leg_2)
  MATLAB Function/1(y) -> foot positions/1

== system Simplified_TriPed/TriPed/World to Robot (Variant) ==
  note: 1) Add Subsystem or Model blocks as valid variant choices.
      | 2) You cannot connect blocks at this level. At simulation, connectivity is automatically
      | determined, based on the active variant and port name matching.
  Free : Subsystem  VariantControl=Choice_2
  Rigid : Subsystem  VariantControl=(default)
  Connection Port : PMIOPort  Side=Left
  Connection Port1 : PMIOPort  Port=2  Side=Right

== system Simplified_TriPed/spider step/Signal Builder ==
  Demux : Demux  Tag=STV Demux  Outputs=1
      settings: DisplayOption=none
  FromWs : FromWorkspace  Tag=STV FromWs  VariableName=tuvar
      SigBuilderData=|
      | common.afterFinalStr = 'Extrapolate'
      | common.sampleTime = 0
      | dataSet.timeRange = [0 10]
      | dataSet.name = 'Group 1'
      | sbobj.Groups.Name = 'Group 1'
      | sbobj.Groups.Signals.Name = 'Signal 1'
      | sbobj.Groups.Signals.XData = [0 0.039788735773 0.0795774715459 0.119366207319 0.159154943092 0.198943678865 0.238732414638 0.278521150411 0.318309886184 0.358098621957 0.39788735773 0.437676093503 0.477464829276 0.5]
      | sbobj.Groups.Signals.YData = [0 0.384 0.38 0.254 0.138 0.064 0.02 0.002 0 0 0.002 0 2.44929359829e-17 0]
      | sbobj.Groups.TimeRange = [0 0.5]
  Signal 1 : Outport  Tag=STV Outport
  wires:
  FromWs/1 -> Demux/1
  Demux/1 -> Signal 1/1

== system Simplified_TriPed/spider step/leg 0 ==
  In1 : Inport
  In2 : Inport  Port=2
  In3 : Inport  Port=3
  Add : Sum
  Add1 : Sum
  Add10 : Sum
  Constant10 : Constant  Value=-0.6
  Constant3 : Constant  Value=0.405
  Constant5 : Constant  Value=0
  Out1 : Outport
  Out2 : Outport  Port=2
  Out3 : Outport  Port=3
  wires:
  Add1/1 -> Out2/1
  Constant5/1 -> Add1/2
  Constant10/1 -> Add10/2
  Add10/1 -> Out3/1
  In2/1 -> Add1/1
  Constant3/1 -> Add/2
  Add/1 -> Out1/1
  In3/1 -> Add10/1
  In1/1 -> Add/1

== system Simplified_TriPed/spider step/leg 1 ==
  In1 : Inport
  In2 : Inport  Port=2
  In3 : Inport  Port=3
  Add2 : Sum
  Add3 : Sum
  Add9 : Sum
  Constant6 : Constant  Value=-0.2025
  Constant7 : Constant  Value=-0.6
  Constant8 : Constant  Value=-0.35074
  Out1 : Outport
  Out2 : Outport  Port=2
  Out3 : Outport  Port=3
  wires:
  In3/1 -> Add9/1
  Constant6/1 -> Add2/2
  Add9/1 -> Out3/1
  Add2/1 -> Out1/1
  Constant8/1 -> Add3/2
  Constant7/1 -> Add9/2
  Add3/1 -> Out2/1
  In2/1 -> Add3/1
  In1/1 -> Add2/1

== system Simplified_TriPed/spider step/leg 2 ==
  In1 : Inport
  In2 : Inport  Port=2
  In3 : Inport  Port=3
  Add4 : Sum
  Add5 : Sum
  Add8 : Sum
  Constant11 : Constant  Value=0.35074
  Constant4 : Constant  Value=-0.6
  Constant9 : Constant  Value=-0.2025
  Out1 : Outport
  Out2 : Outport  Port=2
  Out3 : Outport  Port=3
  wires:
  In2/1 -> Add5/1
  Constant11/1 -> Add5/2
  In3/1 -> Add8/1
  Constant9/1 -> Add4/2
  Add5/1 -> Out2/1
  Add8/1 -> Out3/1
  Constant4/1 -> Add8/2
  Add4/1 -> Out1/1
  In1/1 -> Add4/1

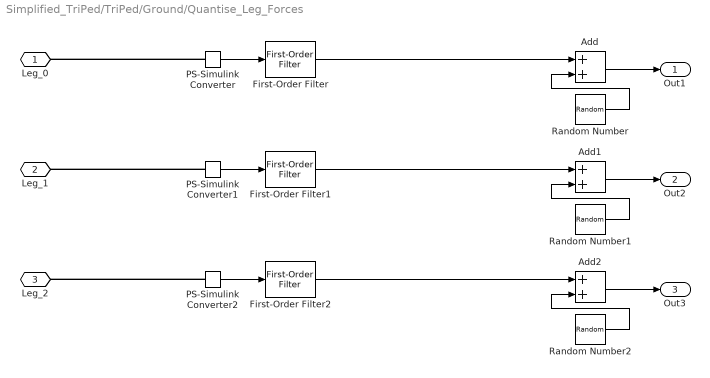
== system Simplified_TriPed/TriPed/Ground/Quantise_Leg_Forces ==
  Add : Sum
  Add1 : Sum
  Add2 : Sum
  First-Order Filter : powerlib_meascontrol/Filters/First-Order Filter  FilterType=Lowpass  Tc=1/10  Ts=0  Initialize=on  Vac_Init=[0, 0, 60]  Vdc_Init=0  PlotResponse=off  FreqRange="[0,  200,  1]"
  First-Order Filter1 : powerlib_meascontrol/Filters/First-Order Filter  FilterType=Lowpass  Tc=1/10  Ts=0  Initialize=on  Vac_Init=[0, 0, 60]  Vdc_Init=0  PlotResponse=off  FreqRange="[0,  200,  1]"
  First-Order Filter2 : powerlib_meascontrol/Filters/First-Order Filter  FilterType=Lowpass  Tc=1/10  Ts=0  Initialize=on  Vac_Init=[0, 0, 60]  Vdc_Init=0  PlotResponse=off  FreqRange="[0,  200,  1]"
  PS-Simulink Converter : nesl_utility/PS-Simulink Converter  PhysicalDomain=network_engine_domain  SubClassName=ps_output  LeftPortType=input  RightPortType=output  PseudoPeriodic=off  Frequencies=[]  Unit=inherit  AffineConversion=off
  PS-Simulink Converter1 : nesl_utility/PS-Simulink Converter  PhysicalDomain=network_engine_domain  SubClassName=ps_output  LeftPortType=input  RightPortType=output  PseudoPeriodic=off  Frequencies=[]  Unit=inherit  AffineConversion=off
  PS-Simulink Converter2 : nesl_utility/PS-Simulink Converter  PhysicalDomain=network_engine_domain  SubClassName=ps_output  LeftPortType=input  RightPortType=output  PseudoPeriodic=off  Frequencies=[]  Unit=inherit  AffineConversion=off
  Random Number : RandomNumber  Mean=1  Variance=0.002^2 /3
  Random Number1 : RandomNumber  Mean=1  Variance=0.002^2 /3
  Random Number2 : RandomNumber  Mean=1  Variance=0.002^2 /3
  Leg_0 : PMIOPort  Side=Left
  Leg_1 : PMIOPort  Port=2  Side=Left
  Leg_2 : PMIOPort  Port=3  Side=Left
  Out1 : Outport
  Out2 : Outport  Port=2
  Out3 : Outport  Port=3
  wires:
  Add/1 -> Out1/1
  Random Number/1 -> Add/2
  PS-Simulink Converter/1 -> First-Order Filter/1
  Random Number1/1 -> Add1/2
  PS-Simulink Converter1/1 -> First-Order Filter1/1
  Add1/1 -> Out2/1
  Random Number2/1 -> Add2/2
  PS-Simulink Converter2/1 -> First-Order Filter2/1
  Add2/1 -> Out3/1
  First-Order Filter/1 -> Add/1
  First-Order Filter1/1 -> Add1/1
  First-Order Filter2/1 -> Add2/1
  connections:
  PS-Simulink Converter/LConn1 -- Leg_0/RConn1
  PS-Simulink Converter1/LConn1 -- Leg_1/RConn1
  PS-Simulink Converter2/LConn1 -- Leg_2/RConn1

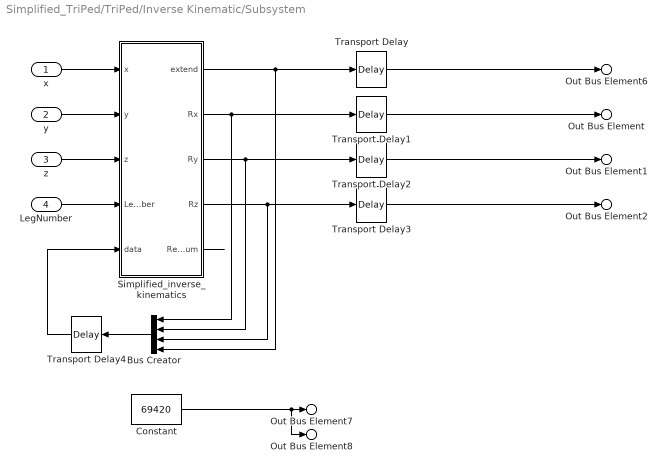
== system Simplified_TriPed/TriPed/Inverse Kinematic/Subsystem ==
  x : Inport
  y : Inport  Port=2
  z : Inport  Port=3
  LegNumber : Inport  Port=4
  Bus Creator : BusCreator  Inputs=4
  Constant : Constant  Value=69420
  Simplified_inverse_kinematics : MATLAB Function  TreatAsAtomicUnit=on
  Transport Delay{,1..3} (4 alike) : TransportDelay  DelayTime=0.01
  Transport Delay4 : TransportDelay  DelayTime=0.001  InitialOutput=[0.0, 0.0000, 0.0, 0]
  Out Bus Element : Outport  PortName=Leg0Bus_OUT  Element=gimbal_joint.Rx
  Out Bus Element1 : Outport  PortName=Leg0Bus_OUT  Element=gimbal_joint.Ry
  Out Bus Element2 : Outport  PortName=Leg0Bus_OUT  Element=gimbal_joint.Rz
  Out Bus Element6 : Outport  PortName=Leg0Bus_OUT  Element=extend_motor.position
  Out Bus Element7 : Outport  PortName=Leg0Bus_OUT  Element=extend_motor.velocity
  Out Bus Element8 : Outport  PortName=Leg0Bus_OUT  Element=extend_motor.effort
  wires:
  y/1 -> Simplified_inverse_kinematics/2(y)
  x/1 -> Simplified_inverse_kinematics/1(x)
  z/1 -> Simplified_inverse_kinematics/3(z)
  Constant/1 -> Out Bus Element8/1, Out Bus Element7/1
  LegNumber/1 -> Simplified_inverse_kinematics/4(LegNumber)
  Simplified_inverse_kinematics/4(Rz) -> Transport Delay3/1, Bus Creator/3
  Simplified_inverse_kinematics/3(Ry) -> Transport Delay2/1, Bus Creator/2
  Simplified_inverse_kinematics/2(Rx) -> Transport Delay1/1, Bus Creator/1
  Bus Creator/1 -> Transport Delay4/1
  Transport Delay4/1 -> Simplified_inverse_kinematics/5(data)
  Simplified_inverse_kinematics/5(Residuum) -> ?
  Simplified_inverse_kinematics/1(extend) -> Transport Delay/1, Bus Creator/4
  Transport Delay/1 -> Out Bus Element6/1
  Transport Delay1/1 -> Out Bus Element/1
  Transport Delay2/1 -> Out Bus Element1/1
  Transport Delay3/1 -> Out Bus Element2/1

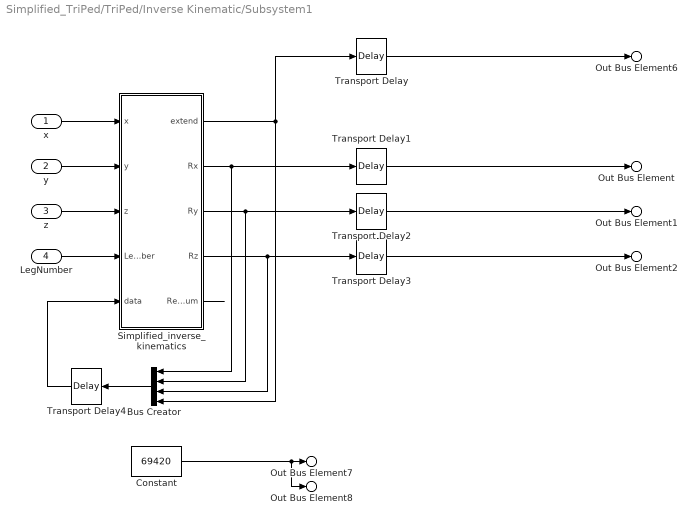
== system Simplified_TriPed/TriPed/Inverse Kinematic/Subsystem1 ==
  x : Inport
  y : Inport  Port=2
  z : Inport  Port=3
  LegNumber : Inport  Port=4
  Bus Creator : BusCreator  Inputs=4
  Constant : Constant  Value=69420
  Simplified_inverse_kinematics : MATLAB Function  TreatAsAtomicUnit=on
  Transport Delay{,1..3} (4 alike) : TransportDelay  DelayTime=0.01
  Transport Delay4 : TransportDelay  DelayTime=0.001  InitialOutput=[0.0, 0.0000, 0.0, 0]
  Out Bus Element : Outport  PortName=Leg0Bus_OUT  Element=gimbal_joint.Rx
  Out Bus Element1 : Outport  PortName=Leg0Bus_OUT  Element=gimbal_joint.Ry
  Out Bus Element2 : Outport  PortName=Leg0Bus_OUT  Element=gimbal_joint.Rz
  Out Bus Element6 : Outport  PortName=Leg0Bus_OUT  Element=extend_motor.position
  Out Bus Element7 : Outport  PortName=Leg0Bus_OUT  Element=extend_motor.velocity
  Out Bus Element8 : Outport  PortName=Leg0Bus_OUT  Element=extend_motor.effort
  wires:
  Transport Delay1/1 -> Out Bus Element/1
  Transport Delay/1 -> Out Bus Element6/1
  Bus Creator/1 -> Transport Delay4/1
  y/1 -> Simplified_inverse_kinematics/2(y)
  Simplified_inverse_kinematics/3(Ry) -> Transport Delay2/1, Bus Creator/2
  Transport Delay3/1 -> Out Bus Element2/1
  Simplified_inverse_kinematics/2(Rx) -> Transport Delay1/1, Bus Creator/1
  x/1 -> Simplified_inverse_kinematics/1(x)
  Simplified_inverse_kinematics/4(Rz) -> Transport Delay3/1, Bus Creator/3
  z/1 -> Simplified_inverse_kinematics/3(z)
  LegNumber/1 -> Simplified_inverse_kinematics/4(LegNumber)
  Transport Delay2/1 -> Out Bus Element1/1
  Transport Delay4/1 -> Simplified_inverse_kinematics/5(data)
  Simplified_inverse_kinematics/1(extend) -> Transport Delay/1, Bus Creator/4
  Simplified_inverse_kinematics/5(Residuum) -> ?
  Constant/1 -> Out Bus Element8/1, Out Bus Element7/1

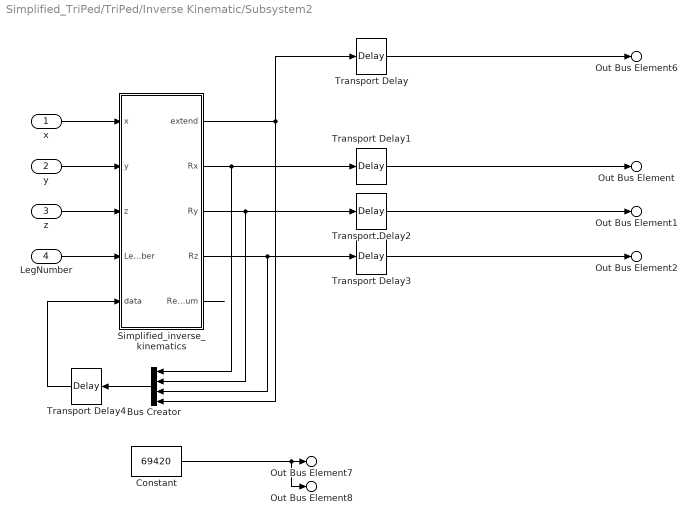
== system Simplified_TriPed/TriPed/Inverse Kinematic/Subsystem2 ==
  x : Inport
  y : Inport  Port=2
  z : Inport  Port=3
  LegNumber : Inport  Port=4
  Bus Creator : BusCreator  Inputs=4
  Constant : Constant  Value=69420
  Simplified_inverse_kinematics : MATLAB Function  TreatAsAtomicUnit=on
  Transport Delay{,1..3} (4 alike) : TransportDelay  DelayTime=0.01
  Transport Delay4 : TransportDelay  DelayTime=0.001  InitialOutput=[0.0, 0.0000, 0.0, 0]
  Out Bus Element : Outport  PortName=Leg0Bus_OUT  Element=gimbal_joint.Rx
  Out Bus Element1 : Outport  PortName=Leg0Bus_OUT  Element=gimbal_joint.Ry
  Out Bus Element2 : Outport  PortName=Leg0Bus_OUT  Element=gimbal_joint.Rz
  Out Bus Element6 : Outport  PortName=Leg0Bus_OUT  Element=extend_motor.position
  Out Bus Element7 : Outport  PortName=Leg0Bus_OUT  Element=extend_motor.velocity
  Out Bus Element8 : Outport  PortName=Leg0Bus_OUT  Element=extend_motor.effort
  wires:
  Transport Delay1/1 -> Out Bus Element/1
  Transport Delay/1 -> Out Bus Element6/1
  Bus Creator/1 -> Transport Delay4/1
  y/1 -> Simplified_inverse_kinematics/2(y)
  Simplified_inverse_kinematics/3(Ry) -> Transport Delay2/1, Bus Creator/2
  Transport Delay3/1 -> Out Bus Element2/1
  Simplified_inverse_kinematics/2(Rx) -> Transport Delay1/1, Bus Creator/1
  x/1 -> Simplified_inverse_kinematics/1(x)
  Simplified_inverse_kinematics/4(Rz) -> Transport Delay3/1, Bus Creator/3
  z/1 -> Simplified_inverse_kinematics/3(z)
  LegNumber/1 -> Simplified_inverse_kinematics/4(LegNumber)
  Transport Delay2/1 -> Out Bus Element1/1
  Transport Delay4/1 -> Simplified_inverse_kinematics/5(data)
  Simplified_inverse_kinematics/1(extend) -> Transport Delay/1, Bus Creator/4
  Simplified_inverse_kinematics/5(Residuum) -> ?
  Constant/1 -> Out Bus Element8/1, Out Bus Element7/1

== system Simplified_TriPed/TriPed/World to Robot (Variant)/Free ==
  World_to_CCS_6-DOF-Joint : sm_lib/Joints/6-DOF Joint  Commented=on  JointMode=Normal  SenseConstraintForce=off  SenseConstraintForceX=off  SenseConstraintForceY=off  SenseConstraintForceZ=off  SenseConstraintTorque=off  SenseConstraintTorqueX=off  SenseConstraintTorqueY=off  SenseConstraintTorqueZ=off  SenseTotalForce=off  SenseTotalForceX=off  SenseTotalForceY=off  SenseTotalForceZ=off  SenseTotalTorque=off  SenseTotalTorqueX=off  SenseTotalTorqueY=off  SenseTotalTorqueZ=off  CompositeWrenchDir=FollowerOnBase  CompositeWrenchFrame=BaseFrame  PxEquilibriumPosition=0  PxEquilibriumPositionUnits=m  PxSpringStiffness=0  PxSpringStiffnessUnits=N/m  PxDampingCoefficient=0  PxDampingCoefficientUnits=N/(m/s)  PxTorqueActuationMode=NoTorque  PxMotionActuationMode=ComputedMotion  PxSensePosition=off  PxSenseVelocity=off  PxSenseAcceleration=off  PxSenseTorqueForce=off  PxSenseLowerLimitTorqueForce=off  PxSenseUpperLimitTorqueForce=off  PxLowerLimitSpecify=off  PxLowerLimitBound=-1  PxLowerLimitBoundUnits=m  PxLowerLimitStiffness=1e6  PxLowerLimitStiffnessUnits=N/m  PxLowerLimitDamping=1e3  PxLowerLimitDampingUnits=N/(m/s)  PxLowerLimitTransitionRegionWidth=1e-4  PxLowerLimitTransitionRegionWidthUnits=m  PxUpperLimitSpecify=off  PxUpperLimitBound=1  PxUpperLimitBoundUnits=m  PxUpperLimitStiffness=1e6  PxUpperLimitStiffnessUnits=N/m  PxUpperLimitDamping=1e3  PxUpperLimitDampingUnits=N/(m/s)  PxUpperLimitTransitionRegionWidth=1e-4  PxUpperLimitTransitionRegionWidthUnits=m  PxPositionTargetSpecify=off  PxPositionTargetPriority=High  PxPositionTargetValue=0  PxPositionTargetValueUnits=m  PxVelocityTargetSpecify=off  PxVelocityTargetPriority=High  PxVelocityTargetValue=0  PxVelocityTargetValueUnits=m/s  PyEquilibriumPosition=0  PyEquilibriumPositionUnits=m  PySpringStiffness=0  PySpringStiffnessUnits=N/m  PyDampingCoefficient=0  PyDampingCoefficientUnits=N/(m/s)  PyTorqueActuationMode=NoTorque  PyMotionActuationMode=ComputedMotion  PySensePosition=off  PySenseVelocity=off  PySenseAcceleration=off  PySenseTorqueForce=off  PySenseLowerLimitTorqueForce=off  PySenseUpperLimitTorqueForce=off  PyLowerLimitSpecify=off  PyLowerLimitBound=-1  PyLowerLimitBoundUnits=m  PyLowerLimitStiffness=1e6  PyLowerLimitStiffnessUnits=N/m  PyLowerLimitDamping=1e3  PyLowerLimitDampingUnits=N/(m/s)  PyLowerLimitTransitionRegionWidth=1e-4  PyLowerLimitTransitionRegionWidthUnits=m  PyUpperLimitSpecify=off  PyUpperLimitBound=1  PyUpperLimitBoundUnits=m  PyUpperLimitStiffness=1e6  PyUpperLimitStiffnessUnits=N/m  PyUpperLimitDamping=1e3  PyUpperLimitDampingUnits=N/(m/s)  PyUpperLimitTransitionRegionWidth=1e-4  PyUpperLimitTransitionRegionWidthUnits=m  PyPositionTargetSpecify=off  PyPositionTargetPriority=High  PyPositionTargetValue=0  PyPositionTargetValueUnits=m  PyVelocityTargetSpecify=off  PyVelocityTargetPriority=High  PyVelocityTargetValue=0  PyVelocityTargetValueUnits=m/s  PzEquilibriumPosition=0  PzEquilibriumPositionUnits=m  PzSpringStiffness=0  PzSpringStiffnessUnits=N/m  PzDampingCoefficient=0  PzDampingCoefficientUnits=N/(m/s)  PzTorqueActuationMode=NoTorque  PzMotionActuationMode=ComputedMotion  PzSensePosition=off  PzSenseVelocity=off  PzSenseAcceleration=off  PzSenseTorqueForce=off  PzSenseLowerLimitTorqueForce=off  PzSenseUpperLimitTorqueForce=off  PzLowerLimitSpecify=off  PzLowerLimitBound=-1  PzLowerLimitBoundUnits=m  PzLowerLimitStiffness=1e6  PzLowerLimitStiffnessUnits=N/m  PzLowerLimitDamping=1e3  PzLowerLimitDampingUnits=N/(m/s)  PzLowerLimitTransitionRegionWidth=1e-4  PzLowerLimitTransitionRegionWidthUnits=m  PzUpperLimitSpecify=off  PzUpperLimitBound=1  PzUpperLimitBoundUnits=m  PzUpperLimitStiffness=1e6  PzUpperLimitStiffnessUnits=N/m  PzUpperLimitDamping=1e3  PzUpperLimitDampingUnits=N/(m/s)  PzUpperLimitTransitionRegionWidth=1e-4  PzUpperLimitTransitionRegionWidthUnits=m  PzPositionTargetSpecify=off  PzPositionTargetPriority=High  PzPositionTargetValue=0  PzPositionTargetValueUnits=m  PzVelocityTargetSpecify=off  PzVelocityTargetPriority=High  PzVelocityTargetValue=0  PzVelocityTargetValueUnits=m/s  SphDefPosRotationMethod=None  SphDefPosRotationAngleUnits=deg  SphDefPosRotationStandardAxis=+Z  SphDefPosRotationAngle=0.0  SphDefPosRotationArbitraryAxis=[0 0 1]  SphDefPosFollAlignAxisA=+X  SphDefPosBaseAlignAxisA=+Y  SphDefPosFollAlignAxisB=+Y  SphDefPosBaseAlignAxisB=+Z  SphDefPosRotationSequenceAxes=FollowerAxes  SphDefPosRotationSequence=XYX  SphDefPosRotationSequenceAngles=[0 0 0]  SphDefPosRotationSequenceAnglesUnits=deg  SphDefPosRotationMatrix=[1 0 0; 0 1 0; 0 0 1]  SphEqPosRotationMethod=None  SphEqPosRotationAngleUnits=deg  SphEqPosRotationStandardAxis=+Z  SphEqPosRotationAngle=0.0  SphEqPosRotationArbitraryAxis=[0 0 1]  SphEqPosFollAlignAxisA=+X  SphEqPosBaseAlignAxisA=+Y  SphEqPosFollAlignAxisB=+Y  SphEqPosBaseAlignAxisB=+Z  SphEqPosRotationSequenceAxes=FollowerAxes  SphEqPosRotationSequence=XYX  SphEqPosRotationSequenceAngles=[0 0 0]  SphEqPosRotationSequenceAnglesUnits=deg  SphEqPosRotationMatrix=[1 0 0; 0 1 0; 0 0 1]  SphSpringStiffness=0  SphSpringStiffnessUnits=N*m/deg  SphDampingCoefficient=0  SphDampingCoefficientUnits=N*m/(deg/s)  SphActuateTorqueX=off  SphActuateTorqueY=off  SphActuateTorqueZ=off  SphActuateTorque=off  SphTorqueActuationMode=NoTorque  SphMotionActuationMode=ComputedMotion  SphActuationFrame=BaseFrame  SphSensePosition=off  SphSenseVelocityX=off  SphSenseVelocityY=off  SphSenseVelocityZ=off  SphSenseVelocity=off  SphSenseAccelerationX=off  SphSenseAccelerationY=off  SphSenseAccelerationZ=off  SphSenseAcceleration=off  SphSenseTorqueX=off  SphSenseTorqueY=off  SphSenseTorqueZ=off  SphSenseTorqueForce=off  SphSenseLowerLimitTorqueMag=off  SphSenseUpperLimitTorqueMag=off  SphSensingFrame=BaseFrame  SphLowerLimitSpecify=off  SphLowerLimitBound=15  SphLowerLimitBoundUnits=deg  SphLowerLimitStiffness=1e4  SphLowerLimitStiffnessUnits=N*m/deg  SphLowerLimitDamping=10  SphLowerLimitDampingUnits=N*m/(deg/s)  SphLowerLimitTransitionRegionWidth=0.1  SphLowerLimitTransitionRegionWidthUnits=deg  SphUpperLimitSpecify=off  SphUpperLimitBound=45  SphUpperLimitBoundUnits=deg  SphUpperLimitStiffness=1e4  SphUpperLimitStiffnessUnits=N*m/deg  SphUpperLimitDamping=10  SphUpperLimitDampingUnits=N*m/(deg/s)  SphUpperLimitTransitionRegionWidth=0.1  SphUpperLimitTransitionRegionWidthUnits=deg  SphPositionTargetRotationMethod=None  SphPositionTargetRotationAngleUnits=deg  SphPositionTargetRotationStandardAxis=+Z  SphPositionTargetRotationAngle=0.0  SphPositionTargetRotationArbitraryAxis=[0 0 1]  SphPositionTargetFollAlignAxisA=+X  SphPositionTargetBaseAlignAxisA=+Y  SphPositionTargetFollAlignAxisB=+Y  SphPositionTargetBaseAlignAxisB=+Z  SphPositionTargetRotationSequenceAxes=FollowerAxes  SphPositionTargetRotationSequence=XYX  SphPositionTargetRotationSequenceAngles=[0 0 0]  SphPositionTargetRotationSequenceAnglesUnits=deg  SphPositionTargetRotationMatrix=[1 0 0; 0 1 0; 0 0 1]  SphPositionTargetSpecify=off  SphPositionTargetPriority=High  SphVelocityTargetValue=[0 0 0]  SphVelocityTargetValueUnits=deg/s  SphVelocityTargetSpecify=off  SphVelocityTargetPriority=High  SphVelocityTargetInFollowerFrame=on
  Connection Port : PMIOPort  Side=Left
  Connection Port1 : PMIOPort  Port=2  Side=Right
  connections:
  World_to_CCS_6-DOF-Joint/RConn1 -- Connection Port1/RConn1
  World_to_CCS_6-DOF-Joint/LConn1 -- Connection Port/RConn1

== system Simplified_TriPed/TriPed/World to Robot (Variant)/Rigid ==
  World_to_CCS : sm_lib/Joints/Weld Joint  JointMode=Normal  SenseConstraintForce=off  SenseConstraintForceX=off  SenseConstraintForceY=off  SenseConstraintForceZ=off  SenseConstraintTorque=off  SenseConstraintTorqueX=off  SenseConstraintTorqueY=off  SenseConstraintTorqueZ=off  SenseTotalForce=off  SenseTotalForceX=off  SenseTotalForceY=off  SenseTotalForceZ=off  SenseTotalTorque=off  SenseTotalTorqueX=off  SenseTotalTorqueY=off  SenseTotalTorqueZ=off  CompositeWrenchDir=FollowerOnBase  CompositeWrenchFrame=BaseFrame
  Connection Port : PMIOPort  Side=Left
  Connection Port1 : PMIOPort  Port=2  Side=Right
  connections:
  World_to_CCS/RConn1 -- Connection Port1/RConn1
  Connection Port/RConn1 -- World_to_CCS/LConn1

== matlab function Simplified_TriPed/Full Body orientation and height control/fullbody kinematics ==
  data: foot0 input; res output; foot1 input; foot2 input; roll input; pitch input; yaw input; height input
function res  = fcn(foot0,foot1,foot2,roll,pitch,yaw,height)
floor_ccs_trafo=transform_to_floor(roll,pitch,yaw,height);

ccs_foot0=floor_ccs_trafo*makehomogenous(foot0);
ccs_foot1=floor_ccs_trafo*makehomogenous(foot1);
ccs_foot2=floor_ccs_trafo*makehomogenous(foot2);
res=[ccs_foot0(1:3);ccs_foot1(1:3);ccs_foot2(1:3)];
end


function [transfM] = transform_to_floor(roll,pitch,yaw,height)
%first translate frame by [x,y,z]
transfM1 = homogenTranslationMat(0,0,-height);
%then rotate using the roll-pitch-yaw convention
transfM2 = makeRotHomogen(eul2rotm([-roll,-pitch,-yaw],'XYZ'));
transfM = transfM1 * transfM2;
end

function [res] = makehomogenous(vector)
    res = [vector(1);vector(2);vector(3);1];
end

function [res] = homogenTranslationMat(x,y,z)
    %this function forms a Translation about a vector x,y,z in a homogenous
    %transformation matrix res. 
    res = [1 0 0 x; 0 1 0 y; 0 0 1 z; 0 0 0 1];
end

function [res] = makeRotHomogen(R)
% this function fills a Rotationmatrix to make it a homogen transformation
% matrix
res = [R(1,1) R(1,2) R(1,3) 0; R(2,1) R(2,2) R(2,3) 0; R(3,1) R(3,2) R(3,3) 0; 0 0 0 1];
end
